simulink model "TrapezoidSimulation"  (R2023b)
settings: Solver=ode4  StartTime=0.0  StopTime=15  FixedStep=ts  MaxStep=0.6  RelTol=1e-3
values from neighbouring files (symbols this model uses):
  N = 120    [TrapezoidMain.m]
  p_left = []    [TrapezoidMain.m]
  p_obstacle = [6,-4;13.5,3;20,-2;27,2;33,0]    [TrapezoidMain.m]
  p_right = []    [TrapezoidMain.m]
  potd = zeros(length(p_obstacle(:,1)),2)    [TrapezoidMain.m]
  potl = zeros(length(p_obstacle(:,1)),2)    [TrapezoidMain.m]
  potu = zeros(length(p_obstacle(:,1)),2)    [TrapezoidMain.m]
  ra = 0.5    [TrapezoidMain.m]
  ro = [0.9;0.9;0.9;0.9;0.9]    [TrapezoidMain.m]
  rs = 0.25    [TrapezoidMain.m]
  so = [3*ro(1);5*ro(2);4*ro(3);5*ro(4);3*ro(5)]    [TrapezoidMain.m]
  vline = 2    [TrapezoidMain.m]
  vmax1 = 1.5    [TrapezoidMain.m]
settings Model: Creator=51078  LastModifiedBy=高岩
settings SolverCC: AlgebraicLoopSolver=TrustRegion
settings DataIOCC: ReturnWorkspaceOutputs=off
settings OptimizationCC: ReuseModelBlockBuffer=off
settings DebuggingCC: UnconnectedInputMsg=warning  UnconnectedOutputMsg=warning  UnconnectedLineMsg=warning  ArithmeticOperatorsInVariantConditions=warning
settings ModelReferenceCC: EnableRefExpFcnMdlSchedulingChecks=on
settings SFSimCC: SimUseLocalCustomCode=off  CustomCodeUndefinedFunction=UseInterfaceOnly
settings RTWCC: RTWUseLocalCustomCode=off  DLArmComputeVersion=19.05
settings CodeAppCC: StateflowObjectComments=on

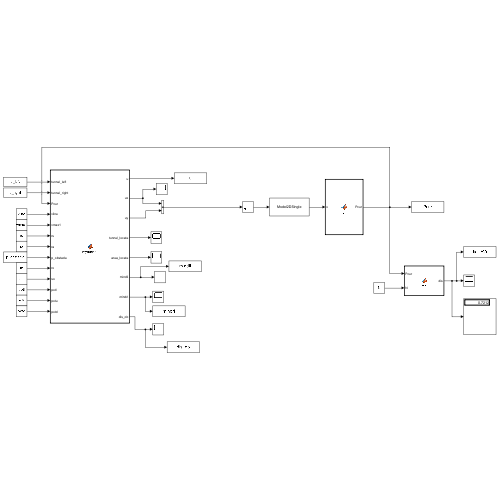
[thumbnail: Simulink's stored preview of the top-level diagram]
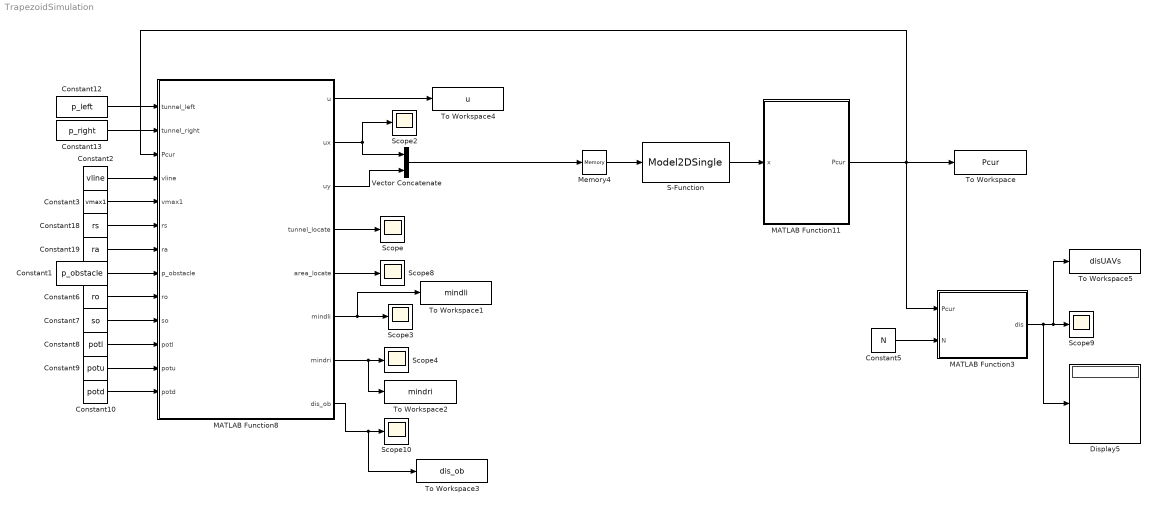
== system TrapezoidSimulation ==
  Constant1 : Constant  Value=p_obstacle
  Constant10 : Constant  Value=potd
  Constant12 : Constant  Value=p_left
  Constant13 : Constant  Value=p_right
  Constant18 : Constant  Value=rs
  Constant19 : Constant  Value=ra
  Constant2 : Constant  Value=vline
  Constant3 : Constant  Value=vmax1
  Constant5 : Constant  Value=N
  Constant6 : Constant  Value=ro
  Constant7 : Constant  Value=so
  Constant8 : Constant  Value=potl
  Constant9 : Constant  Value=potu
  Display5 : Display
  MATLAB Function11 : MATLAB Function  TreatAsAtomicUnit=on
  MATLAB Function3 : MATLAB Function  TreatAsAtomicUnit=on
  MATLAB Function8 : MATLAB Function  TreatAsAtomicUnit=on
  Memory4 : Memory
  S-Function : S-Function  FunctionName=Model2DSingle  SFunctionDeploymentMode=off  EnableBusSupport=off
  Scope{,2..4,8..10} (7 alike) : Scope
  To Workspace : ToWorkspace  VariableName=Pcur  SaveFormat=Timeseries  SampleTime=-1
  To Workspace1 : ToWorkspace  VariableName=mindli  SaveFormat=Timeseries  SampleTime=-1
  To Workspace2 : ToWorkspace  VariableName=mindri  SaveFormat=Timeseries  SampleTime=-1
  To Workspace3 : ToWorkspace  VariableName=dis_ob  SaveFormat=Timeseries  SampleTime=-1
  To Workspace4 : ToWorkspace  VariableName=u  SaveFormat=Timeseries  SampleTime=-1
  To Workspace5 : ToWorkspace  VariableName=disUAVs  SaveFormat=Timeseries  SampleTime=-1
  Vector Concatenate : Concatenate
  wires:
  MATLAB Function8/4(tunnel_locate) -> Scope/1
  Constant12/1 -> MATLAB Function8/1(tunnel_left)
  Constant13/1 -> MATLAB Function8/2(tunnel_right)
  Constant18/1 -> MATLAB Function8/6(rs)
  Constant19/1 -> MATLAB Function8/7(ra)
  MATLAB Function11/1(Pcur) -> MATLAB Function8/3(Pcur), To Workspace/1, MATLAB Function3/1(Pcur)
  MATLAB Function3/1(dis) -> Display5/1, Scope9/1, To Workspace5/1
  Constant5/1 -> MATLAB Function3/2(N)
  Memory4/1 -> S-Function/1
  MATLAB Function8/1(u) -> To Workspace4/1
  S-Function/1 -> MATLAB Function11/1(x)
  MATLAB Function8/3(uy) -> Vector Concatenate/2
  MATLAB Function8/2(ux) -> Scope2/1, Vector Concatenate/1
  Vector Concatenate/1 -> Memory4/1
  Constant2/1 -> MATLAB Function8/4(vline)
  Constant3/1 -> MATLAB Function8/5(vmax1)
  MATLAB Function8/7(mindri) -> To Workspace2/1, Scope4/1
  MATLAB Function8/6(mindli) -> To Workspace1/1, Scope3/1
  MATLAB Function8/5(area_locate) -> Scope8/1
  Constant1/1 -> MATLAB Function8/8(p_obstacle)
  Constant6/1 -> MATLAB Function8/9(ro)
  Constant7/1 -> MATLAB Function8/10(so)
  Constant8/1 -> MATLAB Function8/11(potl)
  Constant9/1 -> MATLAB Function8/12(potu)
  Constant10/1 -> MATLAB Function8/13(potd)
  MATLAB Function8/8(dis_ob) -> To Workspace3/1, Scope10/1

== matlab function TrapezoidSimulation/MATLAB Function3 ==
  data: Pcur input; dis output; N input
function dis = fcn(Pcur,N)
dis=10^5;
for i=1:N
    for j=1:N
        if i~=j
            disij=norm(Pcur(i,1:2) - Pcur(j,1:2));
            if disij<dis
                dis=disij;
            end
        end
    end
end

== matlab function TrapezoidSimulation/MATLAB Function8 ==
  data: tunnel_left input; u output size=[N,2]; ux output; uy output; tunnel_right input; Pcur input; vline input; vmax1 input; rs input; ra input; p_obstacle input; ro input; tunnel_locate output; area_locate output; mindli output; mindri output; so input; potl input; potu input; potd input; dis_ob output
function [u,ux,uy,tunnel_locate,area_locate,mindli,mindri,dis_ob]  = mytunnel(tunnel_left,tunnel_right,Pcur,vline,vmax1,rs,ra,p_obstacle,ro,so,potl,potu,potd)
N=120;

ne=zeros(length(tunnel_left(:,1))-1,2);
nl=zeros(length(tunnel_left(:,1))-1,2);
nr=zeros(length(tunnel_left(:,1))-1,2);
ns=zeros(length(tunnel_left(:,1))-1,2);

c=zeros(length(tunnel_left(:,1))-1,2);
l=zeros(length(tunnel_left(:,1))-1,2);
r=zeros(length(tunnel_left(:,1))-1,2);
s=zeros(length(tunnel_left(:,1))-1,2);


p_fl=zeros(length(tunnel_left(:,1))-1,2);
p_fr=zeros(length(tunnel_left(:,1))-1,2);
p_sl=zeros(length(tunnel_left(:,1))-1,2);
p_sr=zeros(length(tunnel_left(:,1))-1,2);

line_left=diff(tunnel_left);
line_right=diff(tunnel_right);
line_end=tunnel_right(2:end,:)-tunnel_left(2:end,:);
line_start=tunnel_right(1:end-1,:)-tunnel_left(1:end-1,:);


for i=1:length(tunnel_left(:,1))-1
    rot_ne=[0 1;-1 0]; %顺时针90度
    rot_nl=[0 1;-1 0];
    rot_nr=[0 -1;1 0]; %逆时针90度
    rot_ns=[0 -1;1 0];

    A=rot_ne*line_end(i,:)';
    B=rot_nl*line_left(i,:)';
    C=rot_nr*line_right(i,:)';
    D=rot_ns*line_start(i,:)';

    ne(i,:)=(A/norm(A))';
    nl(i,:)=(B/norm(B))';
    nr(i,:)=(C/norm(C))';
    ns(i,:)=(D/norm(D))';

    c(i,:)=line_end(i,:)/norm(line_end(i,:));
    l(i,:)=line_left(i,:)/norm(line_left(i,:));
    r(i,:)=line_right(i,:)/norm(line_right(i,:));
    s(i,:)=line_start(i,:)/norm(line_start(i,:));

end

for j=1:length(tunnel_left(:,1))-1
    p_fl(j,:)=tunnel_left(j+1,:);
    p_fr(j,:)=tunnel_right(j+1,:);
    p_sl(j,:)=tunnel_left(j,:);
    p_sr(j,:)=tunnel_right(j,:);
end

tunnel_locate=zeros(N,1);
area_locate=zeros(N,1);
for i=1:N
    for j=1:length(tunnel_left(:,1))-1
        if dot(nl(j,:),(Pcur(i,1:2)-p_fl(j,:)))>=0 && dot(nr(j,:),(Pcur(i,1:2)-p_fr(j,:)))>=0 ...
                && dot(ne(j,:),(Pcur(i,1:2)-p_fr(j,:)))>=0 && dot(ns(j,:),(Pcur(i,1:2)-p_sr(j,:)))>=0
            tunnel_locate(i)=j;
        end
    end
end

obstalce_locate=zeros(length(p_obstacle(:,1)),1);
for i=1:length(p_obstacle(:,1))
    for j=1:length(tunnel_left(:,1))-1
        if dot(nl(j,:),(p_obstacle(i,:)-p_fl(j,:)))>=0 && dot(nr(j,:),(p_obstacle(i,:)-p_fr(j,:)))>=0 ...
                && dot(ne(j,:),(p_obstacle(i,:)-p_fr(j,:)))>=0 && dot(ns(j,:),(p_obstacle(i,:)-p_sr(j,:)))>=0
            obstalce_locate(i)=j;
        end
    end
end

e1=zeros(N,2);
V1=zeros(N,2);
V2=zeros(N,2);
V3=zeros(N,2);
V4=zeros(N,2);
V5=zeros(N,2);
V6=zeros(N,2);
V=zeros(N,2);
u=zeros(N,2);
dli=zeros(N,1);
dri=zeros(N,1);

alpha=2.5;

dis_ob=10^5;
for i=1:N
    if tunnel_locate(i)~=0
        dli(i) = nl(tunnel_locate(i),:)*(Pcur(i,1:2) -p_fl(tunnel_locate(i),:))';
        dri(i) = nr(tunnel_locate(i),:)*(Pcur(i,1:2) -p_fr(tunnel_locate(i),:))';

        if ((dli(i)>alpha*ra) & (dri(i)>alpha*ra)) || ((dli(i)<alpha*ra) &  (nl(tunnel_locate(i),:)*(-ne(tunnel_locate(i),:))'>=0)) || ((dri(i)<alpha*ra) &  (nr(tunnel_locate(i),:)*(-ne(tunnel_locate(i),:))'>=0))
            e1(i,:)=-ne(tunnel_locate(i),:);
            area_locate(i)=1; %M
        elseif (dli(i)<alpha*ra) &  (nl(tunnel_locate(i),:)*(-ne(tunnel_locate(i),:))'<0)
            aa=mysigma(dli(i),ra,alpha*ra)*(l(tunnel_locate(i),:)+ne(tunnel_locate(i),:))-ne(tunnel_locate(i),:);
            e1(i,:)=aa/norm(aa);
            area_locate(i)=2; %L
        elseif (dri(i)<alpha*ra) &  (nr(tunnel_locate(i),:)*(-ne(tunnel_locate(i),:))'<0)
            bb=mysigma(dri(i),ra,alpha*ra)*(r(tunnel_locate(i),:)+ne(tunnel_locate(i),:))-ne(tunnel_locate(i),:);
            e1(i,:)=bb/norm(bb);
            area_locate(i)=3; %R
        end


        Pt=(ne(tunnel_locate(i),:))'*(ne(tunnel_locate(i),:));

        et=10^(-6);e=10^(-6);k3=1;

        temp = (1+et)*dli(i) - rs*mys(dli(i)/rs,e);
        dVliddli = k3*dmysigma(dli(i),rs,ra)/temp - k3*mysigma(dli(i),rs,ra)*((1+et)-dmys(dli(i)/rs,e))/(temp^2);
        V3(i,:)=((eye(2)-Pt)*(-dVliddli*nl(tunnel_locate(i),:))')';

        temp = (1+et)*dri(i) - rs*mys(dri(i)/rs,e);
        dVriddri = k3*dmysigma(dri(i),rs,ra)/temp - k3*mysigma(dri(i),rs,ra)*((1+et)-dmys(dri(i)/rs,e))/(temp^2);
        V4(i,:)=((eye(2)-Pt)*(-dVriddri*nr(tunnel_locate(i),:))')';
    end

    for j=1:N
        if i~=j
            k2 = 1; e = 0.000001;
            ksimil = (Pcur(i,1:2) - Pcur(j,1:2));
            temp = (1+e)*norm(ksimil) - (2*rs)*mys(norm(ksimil)/(2*rs),e);
            bil = k2*dmysigma(norm(ksimil),2*rs,rs+ra)/temp ...
                - k2*mysigma(norm(ksimil),2*rs,rs+ra)*((1+e)-dmys(norm(ksimil)/(2*rs),e))/(temp^2);
            V2(i,:) = V2(i,:)- bil*(ksimil/norm(ksimil));
        end
    end

    for j=1:length(p_obstacle(:,1))
        k2 = 1; e = 0.000001;
        ksimil = (Pcur(i,1:2) - p_obstacle(j,1:2));
        temp = (1+e)*norm(ksimil) - (rs+ro(j))*mys(norm(ksimil)/(rs+ro(j)),e);
        bil = k2*dmysigma(norm(ksimil),rs+ro(j),ra+ro(j))/temp ...
            - k2*mysigma(norm(ksimil),rs+ro(j),ra+ro(j))*((1+e)-dmys(norm(ksimil)/(rs+ro(j)),e))/(temp^2);
        V5(i,:) = V5(i,:)- bil*(ksimil/norm(ksimil));
    
        if norm(ksimil)<dis_ob
            dis_ob=norm(ksimil);
        end

        if tunnel_locate(i)==obstalce_locate(j)
            if (Pcur(i,:)-p_fl(tunnel_locate(i),:))*(ne(tunnel_locate(i),:))'-(p_obstacle(j,:)-p_fl(tunnel_locate(i),:))*(ne(tunnel_locate(i),:))'<so(j) & (Pcur(i,:)-p_fl(tunnel_locate(i),:))*(ne(tunnel_locate(i),:))'-(p_obstacle(j,:)-p_fl(tunnel_locate(i),:))*(ne(tunnel_locate(i),:))'>-ro(j)
                if (Pcur(i,:)-p_obstacle(j,:))*(c(tunnel_locate(i),:))'<=0

                    rot_nr_obstacle=[0 -1;1 0];%逆时针90度
                    nr_obstacle=(rot_nr_obstacle*(potu(j,:)-potl(j,:))')'/norm(rot_nr_obstacle*(potu(j,:)-potl(j,:))');
                    dri_obstacle = nr_obstacle*(Pcur(i,1:2) -potu(j,:))';

                    et=10^(-6);e=10^(-6);k3=1;
                    Pt=(ne(tunnel_locate(i),:))'*(ne(tunnel_locate(i),:));
                    temp = (1+et)*dri_obstacle - rs*mys(dri_obstacle/rs,e);
                    dVtddri_obstacle = k3*dmysigma(dri_obstacle,rs,ra)/temp - k3*mysigma(dri_obstacle,rs,ra)*((1+et)-dmys(dri_obstacle/rs,e))/(temp^2);
                    V6(i,:)=((eye(2)-Pt)*(-dVtddri_obstacle*nr_obstacle)')';

                    r_obstacle=(potu(j,:)-potl(j,:))/norm(potu(j,:)-potl(j,:));
                    if dri_obstacle<alpha*ra
                        bb=mysigma(dri_obstacle,ra,alpha*ra)*(r_obstacle+ne(tunnel_locate(i),:))-ne(tunnel_locate(i),:);
                        e1(i,:)=bb/norm(bb);
                    end
                elseif (Pcur(i,:)-p_obstacle(j,:))*(c(tunnel_locate(i),:))'>0'

                    rot_nl_obstacle=[0 1;-1 0]; %顺时针90度
                    nl_obstacle=(rot_nl_obstacle*(potd(j,:)-potl(j,:))')'/norm(rot_nl_obstacle*(potd(j,:)-potl(j,:))');
                    dli_obstacle = nl_obstacle*(Pcur(i,1:2) -potd(j,:))';

                    et=10^(-6);e=10^(-6);k3=1;
                    Pt=(ne(tunnel_locate(i),:))'*(ne(tunnel_locate(i),:));
                    temp = (1+et)*dli_obstacle - rs*mys(dli_obstacle/rs,e);
                    dVtddli_obstacle = k3*dmysigma(dli_obstacle,rs,ra)/temp - k3*mysigma(dli_obstacle,rs,ra)*((1+et)-dmys(dli_obstacle/rs,e))/(temp^2);
                    V6(i,:)=((eye(2)-Pt)*(-dVtddli_obstacle*nl_obstacle)')';

                    l_obstacle=(potd(j,:)-potl(j,:))/norm(potd(j,:)-potl(j,:));
                    if dli_obstacle<alpha*ra
                        bb=mysigma(dli_obstacle,ra,alpha*ra)*(l_obstacle+ne(tunnel_locate(i),:))-ne(tunnel_locate(i),:);
                        e1(i,:)=bb/norm(bb);
                    end
                end

            end
        end
    end

    if tunnel_locate(i)==0
         e1(i,:)=[1,0];
    end
    
    V1(i,:) = vline*e1(i,:);

    if isnan(V1(i,1)) || isnan(V1(i,2))
        V1(i,:)=[0,0];
    end
    if isnan(V2(i,1)) || isnan(V2(i,2))
        V2(i,:)=[0,0];
    end
    if isnan(V3(i,1)) || isnan(V3(i,2))
        V3(i,:)=[0,0];
    end
    if isnan(V4(i,1)) || isnan(V4(i,2))
        V4(i,:)=[0,0];
    end
    if isnan(V5(i,1)) || isnan(V5(i,2))
        V5(i,:)=[0,0];
    end
    if isnan(V6(i,1)) || isnan(V6(i,2))
        V6(i,:)=[0,0];
    end

    V(i,:)=V1(i,:)+mysat(V2(i,:)+V3(i,:)+V4(i,:)+V6(i,:),vmax1);
end
mindli=min(dli);
mindri=min(dri);

u=V;
ux = u(:,1);
uy = u(:,2);

== matlab function TrapezoidSimulation/MATLAB Function11 ==
  data: x input; Pcur output size=[N,2]
function Pcur  = fcn(x)
N=120;
Pcur=zeros(N,2);
for i=1:N
    Pcur(i,1)=x(i);
    Pcur(i,2)=x(i+N);
end
end
